simulink model "quxian"  (Simulink 7.6)
settings: Solver=ode4  StartTime=0.0  StopTime=13  FixedStep=0.002  RelTol=1e-3
settings Model: Creator=Tao  LastModifiedBy=Tao

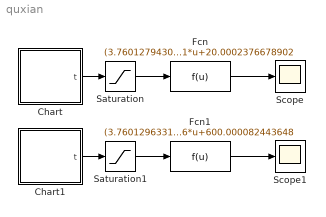
== system quxian ==
  Chart : Stateflow chart  TreatAsAtomicUnit=on
  Chart1 : Stateflow chart  TreatAsAtomicUnit=on
  Fcn : Fcn  Expr=(3.76012794303783e-12)*u^16-(3.77787151438439e-10)*u^15+(1.70366716702520e-08)*u^14-(4.53918294904343e-07)*u^13+(7.91595568148143e-06)*u^12-(9.46991801150381e-05)*u^11+0.000795158956924619*u^10-0.00475883386986616*u^9+0.0207391801532158*u^8-0.0673081776269616*u^7+0.155366359479885*u^6-0.201490925155371*u^5-0.0768516231318135*u^4+2.18034933328387*u^3+0.0584293012534094*u^2-0.00654372848246011*u+20.0002376678902
  Fcn1 : Fcn  Expr=(3.76012963313985e-12)*u^16-(3.44037229998304e-10)*u^15+(1.39996774652558e-08)*u^14-(3.34309394387153e-07)*u^13+(5.21860519506510e-06)*u^12-(5.63398801585665e-05)*u^11+0.000435175092700704*u^10-0.00244274561068785*u^9+0.00982136561852038*u^8-0.0269377658736148*u^7+0.0514170009108526*u^6-0.103245210636221*u^5+0.431283025667506*u^4-2.79148222601809*u^3+0.0172306812740196*u^2-0.00241932536131526*u+600.000082443648
  Saturation : Saturate  UpperLimit=12  LowerLimit=0
  Saturation1 : Saturate  UpperLimit=12  LowerLimit=0
  Scope : Scope
  Scope1 : Scope
      settings: YMin=0  YMax=650
  wires:
  Fcn/1 -> Scope/1
  Chart/1(t) -> Saturation/1
  Saturation/1 -> Fcn/1
  Fcn1/1 -> Scope1/1
  Chart1/1(t) -> Saturation1/1
  Saturation1/1 -> Fcn1/1

== stateflow chart Chart ==
  state on
    en:
    t=0;
  state on2
    en:
    t=t+0.002;
  (default) -> on
  on -> on2
  on2 -> on2
  data: t output double

== stateflow chart Chart1 ==
  state on
    en:
    t=0;
  state on2
    en:
    t=t+0.002;
  (default) -> on
  on -> on2
  on2 -> on2
  data: t output double
